simulink model "SpheroControl_CVT_Comms_LogitechCamera"  (R2014b)
settings: Solver=ode3  StartTime=0.0  StopTime=30  FixedStep=.2  RelTol=1e-3
InitFcn:
  | restartspeed = 65;
  | stopspeed = 1;
  | stopRadius = 25;
  | Kp = 0.2;
  | Ki = 0;
  | Kd = 0;
  | 
  | points = [100, 240; 200, 100; 320, 100; 450, 100; 550, 240];
  | %points = [360, 200];
  | numpoints = size(points, 1);
  | 
  | if ~exist('sph_calibration_angle', 'var')
  | sph_calibration_angle = 0;
  | end
StopFcn:
  | figure;
  | plot(SpheroPos.signals.values(:,1), SpheroPos.signals.values(:, 2), 'kx');
  | hold on;
  | plot(points(:, 1), points(:, 2), 'ro');
  | hold off
  | axis([0 640 0 480])
  | 
  | distEnd =  pdist([points(end, :); SpheroPos.signals.values(end, :)])
undefined symbols (not defined in the file or in its folder): IsPositionTracked, IsSkeletonTracked, JointDepthIndices, JointImageIndices, JointTrackingState, JointWorldCoordinates, none, PositionDepthIndices, PositionImageIndices, PositionWorldCoordinates, SegmentationData, SkeletonTrackingID, videoinput
undefined symbols (not defined in the file): RobotID
libraries: simulink x1, imaqlib x1, aerolibanimutils x1
settings Model: Creator=dsethi  LastModifiedBy=dsethi
settings SolverCC: AlgebraicLoopSolver=LineSearch
settings DataIOCC: SignalLoggingSaveFormat=ModelDataLogs
settings DebuggingCC: MultiTaskDSMMsg=warning  MultiTaskCondExecSysMsg=none
settings RTWCC: IncludeERTFirstTime=on

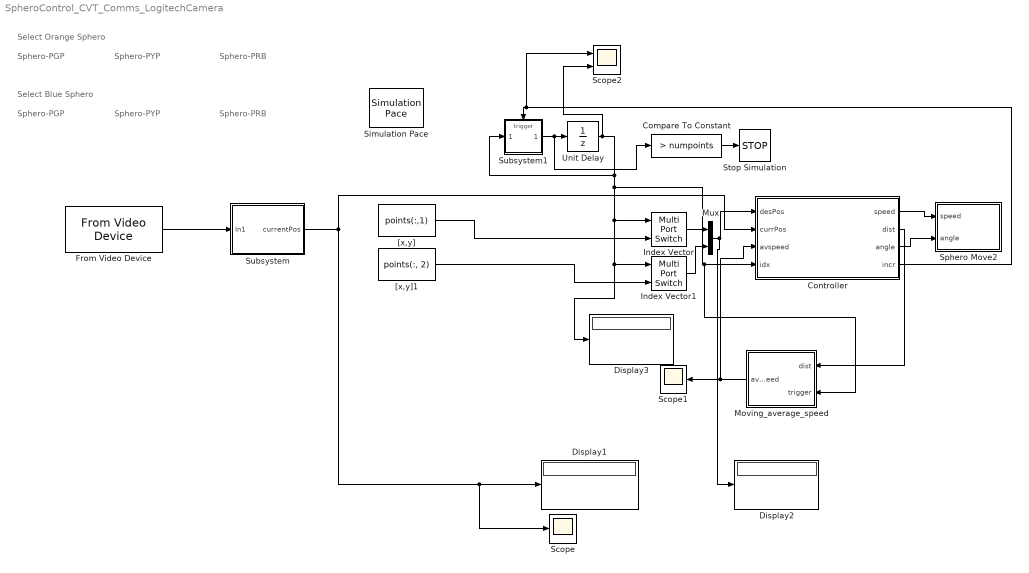
== system SpheroControl_CVT_Comms_LogitechCamera ==
  note: Select Orange Sphero
  note: Sphero-PGP
  note: Sphero-PYP
  note: Sphero-PRB
  note: Select Blue Sphero
  note: Sphero-PGP
  note: Sphero-PYP
  note: Sphero-PRB
  Compare To Constant : simulink/Logic and Bit Operations/Compare To Constant  relop=>  const=numpoints  OutDataTypeStr=boolean
  Controller : Stateflow chart  TreatAsAtomicUnit=on
  Display1 : Display
  Display2 : Display
  Display3 : Display
  From Video Device : imaqlib/From Video Device  DeviceMenu=winvideo 1 (Logitech QuickCam Pro 9000)  Device=winvideo 1 (Logitech QuickCam Pro 9000)  ObjConstructor=videoinput('winvideo', 1)  VideoFormatMenu=RGB24_640x480  VideoFormat=RGB24_640x480  VideoSource=input1  ROIPosition=[0 0 480 640]  EnableHWTrigger=off  TriggerConfiguration=none/none  SampleTime=0.2  OutputPortsMode=One multidimensional signal  DataType=single  CanDoHWTrigger=no  ReturnedColorSpace=rgb  BlockHandle=1921.0006  ROIWidth=640  ROIHeight=480  ROIColumn=0  ROIRow=0  EngXMLPath=E:\jobarchive\R2014bd\2014_07_22_h06m43s29_job123_pass\matlab\toolbox\imaq\imaq\private  DevXMLPath=E:\jobarchive\R2014bd\2014_07_22_h06m43s29_job123_pass\matlab\toolbox\imaq\supportpackages\genericvideo\adaptor\win64  EngLibPath=E:\jobarchive\R2014bd\2014_07_22_h06m43s29_job123_pass\matlab\toolbox\imaq\imaqblks\imaqmex\win64  ColorSpace=rgb  BayerSensorAlignment=grbg  AllMetadata=IsPositionTracked;IsSkeletonTracked;JointDepthIndices;JointImageIndices;JointTrackingState;JointWorldCoordinates;PositionDepthIndices;PositionImageIndices;PositionWorldCoordinates;SegmentationData;SkeletonTrackingID
  Index Vector : MultiPortSwitch  Inputs=1
  Index Vector1 : MultiPortSwitch  Inputs=1
  Moving_average_speed : Subsystem
  Mux : Mux  Inputs=2
  Scope : Scope
      settings: SaveName=SpheroPos
  Scope1 : Scope
      settings: SaveName=movingAvg
  Scope2 : Scope  NumInputPorts=2
      settings: YMin=-5~-5  YMax=5~5  SaveName=movingAvg1
  Simulation Pace : aerolibanimutils/Simulation Pace  SimulationPace=1  SleepMode=MATLAB Thread  OutputPaceError=off  SampleTime=-1
      settings: AttributesFormatString=%<SimulationPace> sec/sec
  Sphero Move2 : MATLAB Function  TreatAsAtomicUnit=on  mask{sphero_RobotID=RobotID.SPHERO_ORANGE}
      mask prompts: sphero_RobotID "Robot"
  Stop Simulation : Stop
  Subsystem : Subsystem  mask{cameraNum=Logitech, desPos=points}
      mask prompts: cameraNum "Camera"; desPos "Desired position (x, y coordinates)"
      mask TypeOptions cameraNum: Logitech | Microsoft
  Subsystem1 : Subsystem
  Unit Delay : UnitDelay  InitialCondition=1  SampleTime=-1
  "[x,y]" : Constant  Value=points(:,1)
  "[x,y]1" : Constant  Value=points(:, 2)
  wires:
  Subsystem/1(currentPos) -> Scope/1, Display1/1, Controller/2(currPos)
  From Video Device/1 -> Subsystem/1(In1)
  Controller/1(speed) -> Sphero Move2/1(speed)
  Controller/3(angle) -> Sphero Move2/2(angle)
  Moving_average_speed/1(avgspeed) -> Scope1/1, Controller/3(avspeed)
  Controller/4(incr) -> Scope2/1, Subsystem1/Trigger
  Subsystem1/1(Out1) -> Compare To Constant/1, Unit Delay/1
  Compare To Constant/1 -> Stop Simulation/1
  Index Vector/1 -> Mux/1
  Index Vector1/1 -> Mux/2
  Mux/1 -> Display2/1, Controller/1(desPos)
  "[x,y]"/1 -> Index Vector/2
  "[x,y]1"/1 -> Index Vector1/2
  Unit Delay/1 -> Scope2/2, Display3/1, Index Vector1/1, Index Vector/1, Moving_average_speed/2(trigger), Controller/4(idx), Subsystem1/1(In1)
  Controller/2(dist) -> Moving_average_speed/1(dist)

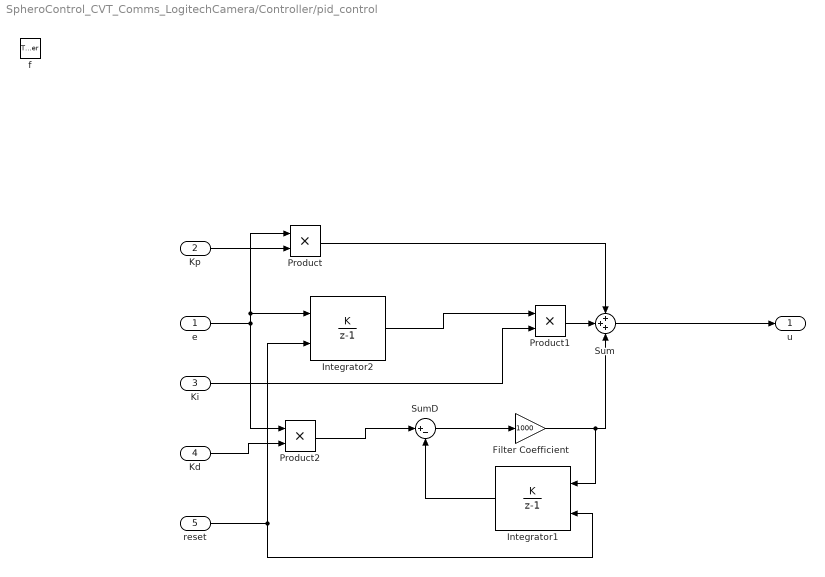
== system SpheroControl_CVT_Comms_LogitechCamera/Controller/pid_control ==
  e : Inport  OutDataTypeStr=double  PortDimensions=1
  Kp : Inport  Port=2  OutDataTypeStr=double  PortDimensions=1
  Ki : Inport  Port=3  OutDataTypeStr=double  PortDimensions=1
  Kd : Inport  Port=4  OutDataTypeStr=double  PortDimensions=1
  reset : Inport  Port=5  OutDataTypeStr=double  PortDimensions=1
  f : TriggerPort  TriggerType=function-call
      settings: CopyFcn=Stateflow.SLINSF.SimulinkMan.removeBlockPreDeleteFcn  PreDeleteFcn=Stateflow.SLINSF.SimulinkMan.unsafePredeleteFcn
  Filter Coefficient : Gain  Gain=1000
  Integrator1 : DiscreteIntegrator  IntegratorMethod=Accumulation: Forward Euler  ExternalReset=rising  InitialConditionSetting=State (most efficient)  SampleTime=-1
  Integrator2 : DiscreteIntegrator  IntegratorMethod=Accumulation: Forward Euler  ExternalReset=rising  InitialConditionSetting=State (most efficient)  SampleTime=-1
  Product : Product
  Product1 : Product
  Product2 : Product
  Sum : Sum  Inputs=+++
  SumD : Sum  DisableCoverage=on  Inputs=|+-
  u : Outport
  wires:
  Sum/1 -> u/1
  Product1/1 -> Sum/2
  Integrator1/1 -> SumD/2
  Filter Coefficient/1 -> Integrator1/1, Sum/3
  SumD/1 -> Filter Coefficient/1
  Product2/1 -> SumD/1
  Product/1 -> Sum/1
  e/1 -> Product/1, Integrator2/1, Product2/1
  Kp/1 -> Product/2
  Integrator2/1 -> Product1/1
  Ki/1 -> Product1/2
  Kd/1 -> Product2/2
  reset/1 -> Integrator1/2, Integrator2/2

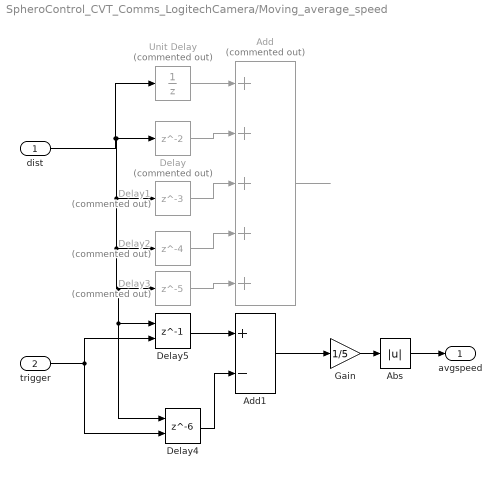
== system SpheroControl_CVT_Comms_LogitechCamera/Moving_average_speed ==
  dist : Inport
  trigger : Inport  Port=2
  Abs : Abs
  Add : Sum  Commented=on  Inputs=+++++
  Add1 : Sum  Inputs=+-
  Delay : Delay  Commented=on
  Delay1 : Delay  Commented=on  DelayLength=3
  Delay2 : Delay  Commented=on  DelayLength=4
  Delay3 : Delay  Commented=on  DelayLength=5
  Delay4 : Delay  DelayLength=6  ExternalReset=Rising
      settings: InputPortMap=u0,r5
  Delay5 : Delay  DelayLength=1  ExternalReset=Rising
      settings: InputPortMap=u0,r5
  Gain : Gain  Gain=1/5
  Unit Delay : UnitDelay  Commented=on  SampleTime=-1
  avgspeed : Outport
  wires:
  Delay/1 -> Add/2
  dist/1 -> Unit Delay/1, Delay4/1, Delay5/1, Delay3/1, Delay2/1, Delay1/1, Delay/1
  Unit Delay/1 -> Add/1
  Delay1/1 -> Add/3
  Delay2/1 -> Add/4
  Delay3/1 -> Add/5
  Add/1 -> ?
  Gain/1 -> Abs/1
  Delay4/1 -> Add1/2
  Add1/1 -> Gain/1
  Delay5/1 -> Add1/1
  Abs/1 -> avgspeed/1
  trigger/1 -> Delay5/2, Delay4/2

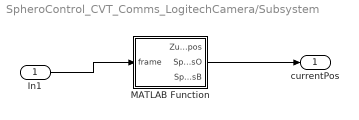
== system SpheroControl_CVT_Comms_LogitechCamera/Subsystem ==
  In1 : Inport
  MATLAB Function : MATLAB Function  TreatAsAtomicUnit=on
  currentPos : Outport
  wires:
  In1/1 -> MATLAB Function/1(frame)
  MATLAB Function/2(SpheroposO) -> currentPos/1

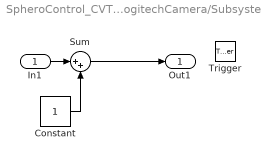
== system SpheroControl_CVT_Comms_LogitechCamera/Subsystem1 ==
  In1 : Inport
  Trigger : TriggerPort  PortDimensions=1
  Constant : Constant
  Sum : Sum  Inputs=|++
  Out1 : Outport  InitialOutput=1
  wires:
  Constant/1 -> Sum/2
  In1/1 -> Sum/1
  Sum/1 -> Out1/1

== matlab function SpheroControl_CVT_Comms_LogitechCamera/Subsystem/MATLAB Function ==
  data: frame input; Zumopos output single; SpheroposO output; SpheroposB output
function [Zumopos, SpheroposO, SpheroposB] = fcn(frame)
%#codegen
persistent init

coder.extrinsic('detectMinions2')

Zumopos = single([0 0]);
SpheroposO = [0; 0];
SpheroposB = [0; 0];

if isempty(init)
    [Zumopos, SpheroposO, SpheroposB] = detectMinions2(frame, 1);
    init = 1;
else
    [Zumopos, SpheropostempO, SpheropostempB] = detectMinions2(frame);
    SpheroposO = SpheropostempO';
    SpheroposB = SpheropostempB';
    
end

== stateflow chart SpheroControl_CVT_Comms_LogitechCamera/Controller ==
  state Control [parallel]
    settings: executionOrder=2
    state Motion
      en, du: speed = pid_control(dist, Kp, Ki, Kd, idx);
    state Stop
      en: incr = 1;
      en, du: speed = 0;
      ex: incr = 0;
    state Restart
      en, du: speed = restartspeed;
    (default) -> Motion : {incr = 0;}
    Stop -> Motion [order 2] : [dist>stopRadius]
    Motion -> Stop [order 1] : [dist<stopRadius]
    Restart -> Motion [order 1] : [avspeed>stopspeed]
    Motion -> Restart [order 2] : [avspeed<stopspeed]
    Restart -> Stop [order 2] : [dist<stopRadius]
    Stop -> Restart [order 1] : [avspeed<stopspeed && dist>stopRadius]
  state ComputeDist [parallel]
    en, du: [dist, angle] = relativePos(desPos, currPos);
    settings: executionOrder=1
  state u = pid_control(e,Kp,Ki,Kd,reset) [function]
  data: desiredPos function_input; currentPos function_input; distance function_output; angleOut function_output; e function_input double size=1; u function_output; Kp function_input double size=1; Ki function_input double size=1; Kd function_input double size=1; reset function_input double size=1; speed output; dist output; angle output; desPos input; currPos input; Kp parameter; Ki parameter; Kd parameter; avspeed input; stopspeed parameter; restartspeed parameter; stopRadius parameter; incr output; idx input
  function [distance, angleOut] = relativePos(desiredPos, currentPos):
    | function [distance, angleOut] = relativePos(desiredPos, currentPos)
    | 
    | coder.extrinsic('radtodeg', 'pdist')
    | distance = 0;
    | angleOut = 0;
    | 
    | if currPos(1)<0 || currPos(2)<0
    |     
    |     return
    | end
    | %% Angle and distance calculation
    |  
    |     %Angle of desired position wrt y axis (or orientation of sphero)
    |     angleOut = atan2(desiredPos(1)-currentPos(1), desiredPos(2)-currentPos(2));
    | 
    |     if angleOut<0
    |         angleOut = -angleOut;
    |     else
    |         angleOut = 2*pi-angleOut;
    |     end
    | 
    |     angleOut = radtodeg(angleOut);
    | 
    |     distance = pdist([desiredPos'; currentPos']); %Distance or the error

== matlab function SpheroControl_CVT_Comms_LogitechCamera/Sphero Move2 ==
  data: speed input; angle input; sphero_RobotID parameter Enum: RobotID
function fcn(speed, angle, sphero_RobotID)
%#codegen
coder.extrinsic('move_sphero_comms')

move_sphero_comms(sphero_RobotID, speed, angle);
